simulink model "analise_pi_d_planta"  (R2025a)
settings: Solver=VariableStepAuto  StartTime=0.0  StopTime=150  RelTol=1e-3
values from neighbouring files (symbols this model uses):
  alpha = 0.1    [simulink_constants.m]
  Delay = 0.1    [simulink_constants.m]
  kp = 10    [simulink_constants.m]
  Np = 10^(-9)    (= 1e-09)    [simulink_constants.m]
  td = 0.05    [simulink_constants.m]
  ti = 0.17    [simulink_constants.m]
  Ts = 0.5    [filtro.m]    (also in simulink_constants.m = 0.02; teste2.m)
libraries: simulink x2, cstblocks x1
settings Model: Creator=joaof  LastModifiedBy=joaof

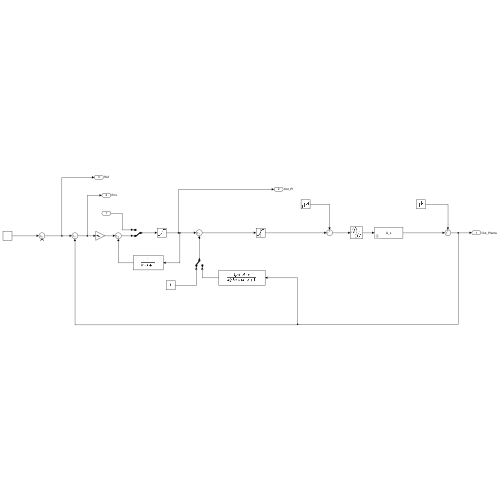
[thumbnail: Simulink's stored preview of the top-level diagram]
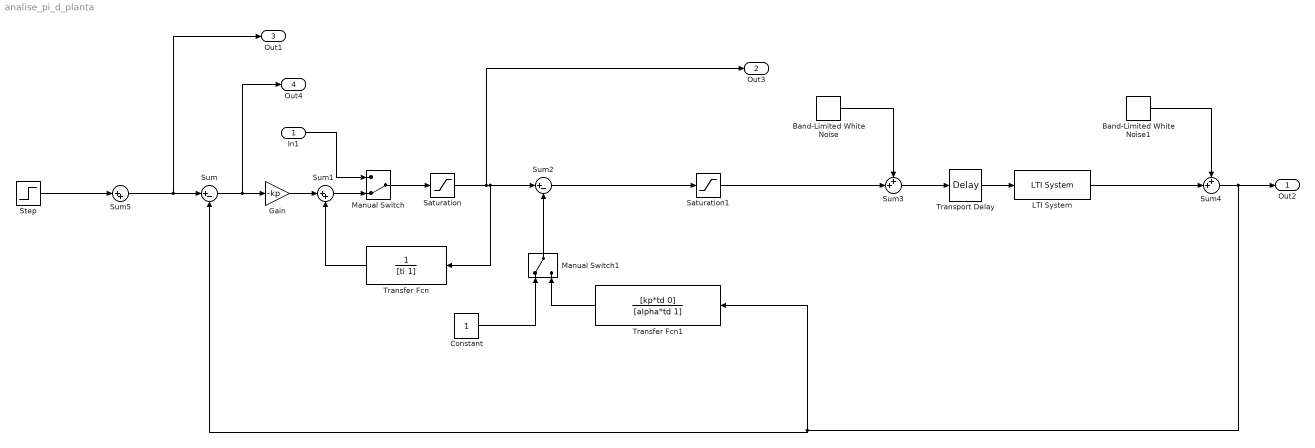
== system analise_pi_d_planta ==
  In1 : Inport
  Band-Limited White Noise : simulink/Sources/Band-Limited White Noise  Cov=[Np]  Ts=Ts  seed=[23341]
  Band-Limited White Noise1 : simulink/Sources/Band-Limited White Noise  Cov=[Np]  Ts=Ts  seed=[23341]
  Constant : Constant
  Gain : Gain  Gain=-kp
  LTI System : cstblocks/LTI System  sys=G_s  IC=[]  PadeOrder=0
  Manual Switch : ManualSwitch  CurrentSetting=0
  Manual Switch1 : ManualSwitch
  Saturation : Saturate  UpperLimit=2  LowerLimit=-2
  Saturation1 : Saturate  UpperLimit=2  LowerLimit=-2
  Step : Step  After=0.18  SampleTime=0
  Sum : Sum  Inputs=|+-
  Sum1 : Sum  Inputs=|++
  Sum2 : Sum  Inputs=|+-
  Sum3 : Sum  Inputs=++|
  Sum4 : Sum  Inputs=++|
  Sum5 : Sum  Inputs=|++
  Transfer Fcn : TransferFcn  Denominator=[ti 1]
  Transfer Fcn1 : TransferFcn  Numerator=[kp*td 0]  Denominator=[alpha*td 1]
  Transport Delay : TransportDelay  DelayTime=Delay
  Out2 : Outport  SignalName=Out_Planta
  Out3 : Outport  Port=2  SignalName=Out_PI
  Out1 : Outport  Port=3  SignalName=Ref
  Out4 : Outport  Port=4  SignalName=Erro
  wires:
  Sum/1 -> Out4/1, Gain/1
  Gain/1 -> Sum1/1
  In1/1 -> Manual Switch/1
  Sum1/1 -> Manual Switch/2
  Manual Switch/1 -> Saturation/1
  Constant/1 -> Manual Switch1/1
  Transfer Fcn1/1 -> Manual Switch1/2
  Manual Switch1/1 -> Sum2/2
  Band-Limited White Noise/1 -> Sum3/1
  Sum3/1 -> Transport Delay/1
  Transport Delay/1 -> LTI System/1
  LTI System/1 -> Sum4/2
  Band-Limited White Noise1/1 -> Sum4/1
  Sum4/1 -> Sum/2, Transfer Fcn1/1, Out2/1
  Sum2/1 -> Saturation1/1
  Saturation/1 -> Out3/1, Transfer Fcn/1, Sum2/1
  Transfer Fcn/1 -> Sum1/2
  Step/1 -> Sum5/1
  Sum5/1 -> Out1/1, Sum/1
  Saturation1/1 -> Sum3/2
